simulink model "Beerbot_Simulink"  (R2020a)
settings: Solver=FixedStepAuto  StartTime=0.0  StopTime=31.5  FixedStep=0.1  RelTol=1e-3
values from neighbouring files (symbols this model uses):
  bot_wheel_distance = 0.5948    [Beerbot.m]    (also in run_Beerbot_Simulink.m)
  dual_wheel_slip_acc_thres = 1.5    [run_Beerbot_Simulink.m]
  heading_initial = Compass_Heading(1)    [run_Beerbot_Simulink.m]
  wheel_slip_detection_thres = 10.15    [run_Beerbot_Simulink.m]
  wheel_slip_detection_thres_factor = 0.8    [run_Beerbot_Simulink.m]
undefined symbols (not defined in the file or in its folder): DiscIntNeverNeededParam, theta_initial
libraries: simulink x10, dspstat3 x5, simulink_extras x2, robotmobilelib x1
settings Model: Creator=Besitzer  LastModifiedBy=Besitzer

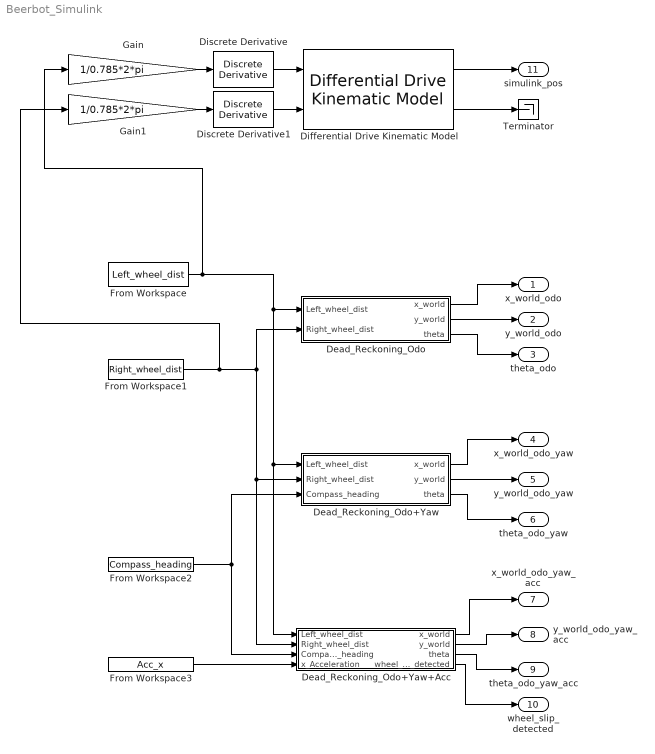
== system Beerbot_Simulink ==
  Dead_Reckoning_Odo : Subsystem
  Dead_Reckoning_Odo+Yaw : Subsystem
  Dead_Reckoning_Odo+Yaw+Acc : Subsystem
  Differential Drive Kinematic Model : robotmobilelib/Differential Drive Kinematic Model  VehicleInputs=Wheel Speeds  WheelRadius=0.1233  WheelSpeedRange=[-inf inf]  TrackWidth=0.585  InitialState=[0; 0; 0.75]  SimulateUsing=Interpreted execution
      settings: SourceProductBaseCode=RO
  Discrete Derivative : simulink/Discrete/Discrete Derivative  gainval=1.0  ICPrevScaledInput=0.0  OutMin=[]  OutMax=[]  OutDataType=fixdt(1, 16)  OutScaling=2^-10  DoSatur=off
  Discrete Derivative1 : simulink/Discrete/Discrete Derivative  gainval=1.0  ICPrevScaledInput=0.0  OutMin=[]  OutMax=[]  OutDataType=fixdt(1, 16)  OutScaling=2^-10  DoSatur=off
  From Workspace : FromWorkspace  VariableName=Left_wheel_dist
  From Workspace1 : FromWorkspace  VariableName=Right_wheel_dist
  From Workspace2 : FromWorkspace  VariableName=Compass_heading
  From Workspace3 : FromWorkspace  VariableName=Acc_x
  Gain : Gain  Gain=1/0.785*2*pi
  Gain1 : Gain  Gain=1/0.785*2*pi
  Terminator : Terminator
  x_world_odo : Outport
  y_world_odo : Outport  Port=2
  theta_odo : Outport  Port=3
  x_world_odo_yaw : Outport  Port=4
  y_world_odo_yaw : Outport  Port=5
  theta_odo_yaw : Outport  Port=6
  x_world_odo_yaw_acc : Outport  Port=7
  y_world_odo_yaw_acc : Outport  Port=8
  theta_odo_yaw_acc : Outport  Port=9
  wheel_slip_detected : Outport  Port=10
  simulink_pos : Outport  Port=11
  wires:
  From Workspace1/1 -> Gain1/1, Dead_Reckoning_Odo+Yaw+Acc/2(Right_wheel_dist), Dead_Reckoning_Odo+Yaw/2(Right_wheel_dist), Dead_Reckoning_Odo/2(Right_wheel_dist)
  Dead_Reckoning_Odo/3(theta) -> theta_odo/1
  Dead_Reckoning_Odo/1(x_world) -> x_world_odo/1
  Dead_Reckoning_Odo/2(y_world) -> y_world_odo/1
  From Workspace2/1 -> Dead_Reckoning_Odo+Yaw+Acc/3(Compass_heading), Dead_Reckoning_Odo+Yaw/3(Compass_heading)
  Dead_Reckoning_Odo+Yaw/1(x_world) -> x_world_odo_yaw/1
  Dead_Reckoning_Odo+Yaw/3(theta) -> theta_odo_yaw/1
  From Workspace3/1 -> Dead_Reckoning_Odo+Yaw+Acc/4(x_Acceleration)
  Dead_Reckoning_Odo+Yaw+Acc/3(theta) -> theta_odo_yaw_acc/1
  Dead_Reckoning_Odo+Yaw+Acc/2(y_world) -> y_world_odo_yaw_acc/1
  Dead_Reckoning_Odo+Yaw+Acc/1(x_world) -> x_world_odo_yaw_acc/1
  Dead_Reckoning_Odo+Yaw/2(y_world) -> y_world_odo_yaw/1
  Dead_Reckoning_Odo+Yaw+Acc/4(wheel_slip_detected) -> wheel_slip_detected/1
  Discrete Derivative/1 -> Differential Drive Kinematic Model/1
  Discrete Derivative1/1 -> Differential Drive Kinematic Model/2
  Differential Drive Kinematic Model/1 -> simulink_pos/1
  Differential Drive Kinematic Model/2 -> Terminator/1
  From Workspace/1 -> Gain/1, Dead_Reckoning_Odo/1(Left_wheel_dist), Dead_Reckoning_Odo+Yaw+Acc/1(Left_wheel_dist), Dead_Reckoning_Odo+Yaw/1(Left_wheel_dist)
  Gain/1 -> Discrete Derivative/1
  Gain1/1 -> Discrete Derivative1/1

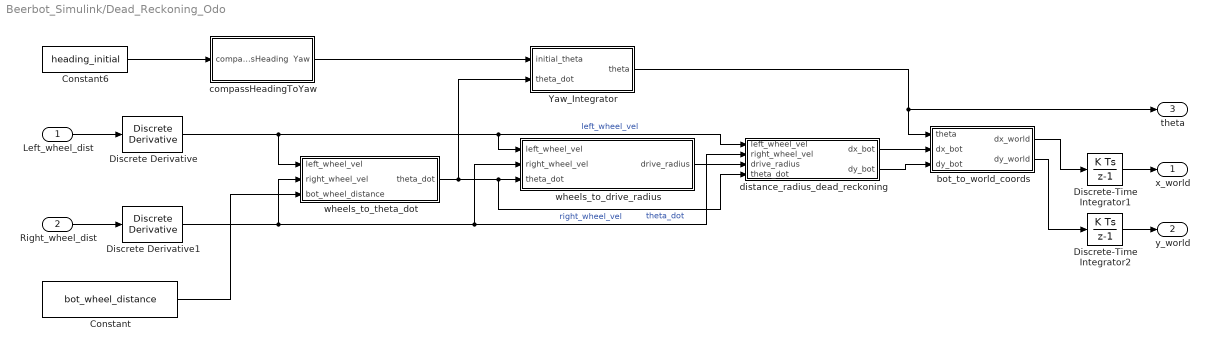
== system Beerbot_Simulink/Dead_Reckoning_Odo ==
  Left_wheel_dist : Inport
  Right_wheel_dist : Inport  Port=2
  Constant : Constant  Value=bot_wheel_distance
  Constant6 : Constant  Value=heading_initial
  Discrete Derivative : simulink/Discrete/Discrete Derivative  gainval=1.0  ICPrevScaledInput=0.0  OutMin=[]  OutMax=[]  OutDataType=fixdt(1, 16)  OutScaling=2^-10  DoSatur=off
      settings: AttributesFormatString=%<Name>
  Discrete Derivative1 : simulink/Discrete/Discrete Derivative  gainval=1.0  ICPrevScaledInput=0.0  OutMin=[]  OutMax=[]  OutDataType=fixdt(1, 16)  OutScaling=2^-10  DoSatur=off
      settings: AttributesFormatString=%<Name>
  Discrete-Time Integrator1 : DiscreteIntegrator  SampleTime=-1  ICPrevOutput=DiscIntNeverNeededParam  ICPrevScaledInput=DiscIntNeverNeededParam
      settings: AttributesFormatString=%<Name>
  Discrete-Time Integrator2 : DiscreteIntegrator  SampleTime=-1  ICPrevOutput=DiscIntNeverNeededParam  ICPrevScaledInput=DiscIntNeverNeededParam
      settings: AttributesFormatString=%<Name>
  Yaw_Integrator : Subsystem
  bot_to_world_coords : Subsystem
  compassHeadingToYaw : Subsystem
  distance_radius_dead_reckoning : Subsystem
  wheels_to_drive_radius : Subsystem
  wheels_to_theta_dot : Subsystem
  x_world : Outport
  y_world : Outport  Port=2
  theta : Outport  Port=3
  wires:
  Left_wheel_dist/1 -> Discrete Derivative/1
  Right_wheel_dist/1 -> Discrete Derivative1/1
  Discrete Derivative1/1 -> wheels_to_theta_dot/2(right_wheel_vel), wheels_to_drive_radius/2(right_wheel_vel), distance_radius_dead_reckoning/2(right_wheel_vel)  "right_wheel_vel"
  Discrete Derivative/1 -> distance_radius_dead_reckoning/1(left_wheel_vel), wheels_to_drive_radius/1(left_wheel_vel), wheels_to_theta_dot/1(left_wheel_vel)  "left_wheel_vel"
  wheels_to_theta_dot/1(theta_dot) -> distance_radius_dead_reckoning/4(theta_dot), wheels_to_drive_radius/3(theta_dot), Yaw_Integrator/2(theta_dot)  "theta_dot"
  Yaw_Integrator/1(theta) -> theta/1, bot_to_world_coords/1(theta)
  Discrete-Time Integrator1/1 -> x_world/1
  Discrete-Time Integrator2/1 -> y_world/1
  compassHeadingToYaw/1(Yaw) -> Yaw_Integrator/1(initial_theta)
  Constant6/1 -> compassHeadingToYaw/1(compassHeading)
  bot_to_world_coords/1(dx_world) -> Discrete-Time Integrator1/1
  bot_to_world_coords/2(dy_world) -> Discrete-Time Integrator2/1
  Constant/1 -> wheels_to_theta_dot/3(bot_wheel_distance)
  wheels_to_drive_radius/1(drive_radius) -> distance_radius_dead_reckoning/3(drive_radius)
  distance_radius_dead_reckoning/1(dx_bot) -> bot_to_world_coords/2(dx_bot)
  distance_radius_dead_reckoning/2(dy_bot) -> bot_to_world_coords/3(dy_bot)

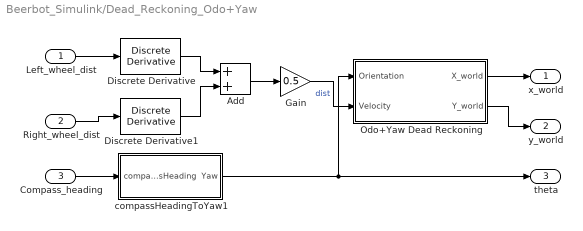
== system Beerbot_Simulink/Dead_Reckoning_Odo+Yaw ==
  Left_wheel_dist : Inport
  Right_wheel_dist : Inport  Port=2
  Compass_heading : Inport  Port=3
  Add : Sum
  Discrete Derivative : simulink/Discrete/Discrete Derivative  gainval=1.0  ICPrevScaledInput=0.0  OutMin=[]  OutMax=[]  OutDataType=fixdt(1, 16)  OutScaling=2^-10  DoSatur=off
  Discrete Derivative1 : simulink/Discrete/Discrete Derivative  gainval=1.0  ICPrevScaledInput=0.0  OutMin=[]  OutMax=[]  OutDataType=fixdt(1, 16)  OutScaling=2^-10  DoSatur=off
  Gain : Gain  Gain=0.5
  Odo+Yaw Dead Reckoning : Subsystem
  compassHeadingToYaw1 : Subsystem
  x_world : Outport
  y_world : Outport  Port=2
  theta : Outport  Port=3
  wires:
  Add/1 -> Gain/1
  Compass_heading/1 -> compassHeadingToYaw1/1(compassHeading)
  compassHeadingToYaw1/1(Yaw) -> Odo+Yaw Dead Reckoning/1(Orientation), theta/1
  Left_wheel_dist/1 -> Discrete Derivative/1
  Discrete Derivative/1 -> Add/1
  Discrete Derivative1/1 -> Add/2
  Right_wheel_dist/1 -> Discrete Derivative1/1
  Gain/1 -> Odo+Yaw Dead Reckoning/2(Velocity)  "dist"
  Odo+Yaw Dead Reckoning/1(X_world) -> x_world/1
  Odo+Yaw Dead Reckoning/2(Y_world) -> y_world/1

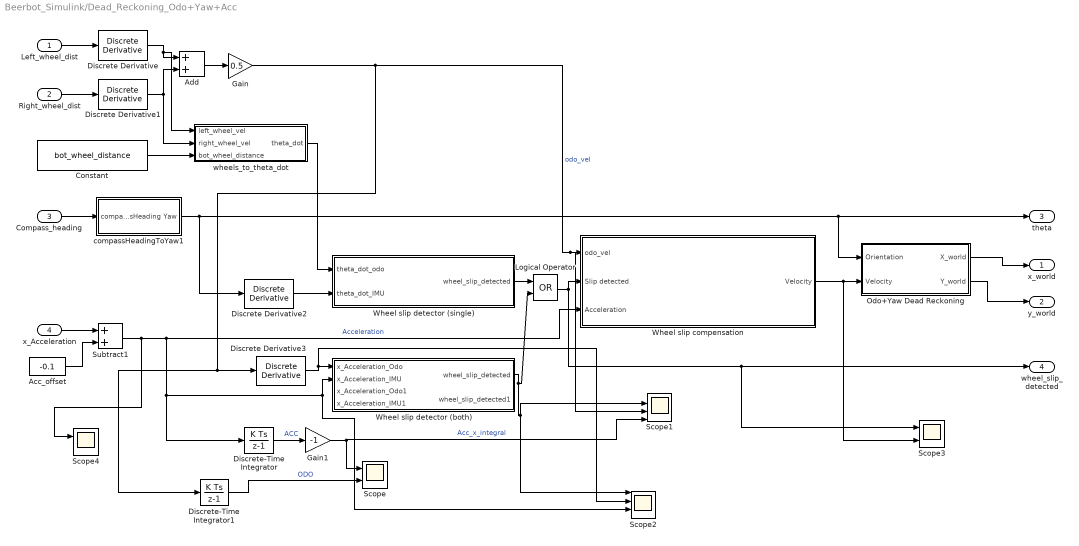
== system Beerbot_Simulink/Dead_Reckoning_Odo+Yaw+Acc ==
  Left_wheel_dist : Inport
  Right_wheel_dist : Inport  Port=2
  Compass_heading : Inport  Port=3
  x_Acceleration : Inport  Port=4
  Acc_offset : Constant  Value=-0.1
  Add : Sum
  Constant : Constant  Value=bot_wheel_distance
  Discrete Derivative{,1..3} (4 alike) : simulink/Discrete/Discrete Derivative  gainval=1.0  ICPrevScaledInput=0.0  OutMin=[]  OutMax=[]  OutDataType=fixdt(1, 16)  OutScaling=2^-10  DoSatur=off
  Discrete-Time Integrator : DiscreteIntegrator  SampleTime=-1  ICPrevOutput=DiscIntNeverNeededParam  ICPrevScaledInput=DiscIntNeverNeededParam
  Discrete-Time Integrator1 : DiscreteIntegrator  SampleTime=-1  ICPrevOutput=DiscIntNeverNeededParam  ICPrevScaledInput=DiscIntNeverNeededParam
  Gain : Gain  Gain=0.5
  Gain1 : Gain  Gain=-1
  Logical Operator : Logic  Operator=OR  AllPortsSameDT=off  OutDataTypeStr=boolean
  Odo+Yaw Dead Reckoning : Subsystem
  Scope : Scope  NumInputPorts=2
  Scope1 : Scope  NumInputPorts=4
  Scope2 : Scope  NumInputPorts=4
  Scope3 : Scope  NumInputPorts=2
  Scope4 : Scope  NumInputPorts=2
  Subtract1 : Sum
  Wheel slip compensation : Subsystem
  Wheel slip detector (both) : Subsystem
  Wheel slip detector (single) : Subsystem
  compassHeadingToYaw1 : Subsystem
  wheels_to_theta_dot : Subsystem
  x_world : Outport
  y_world : Outport  Port=2
  theta : Outport  Port=3
  wheel_slip_detected : Outport  Port=4  OutDataTypeStr=boolean  LockScale=on
  wires:
  Add/1 -> Gain/1
  Compass_heading/1 -> compassHeadingToYaw1/1(compassHeading)
  compassHeadingToYaw1/1(Yaw) -> Discrete Derivative2/1, Odo+Yaw Dead Reckoning/1(Orientation), theta/1
  Left_wheel_dist/1 -> Discrete Derivative/1
  Discrete Derivative/1 -> wheels_to_theta_dot/1(left_wheel_vel), Add/1
  Discrete Derivative1/1 -> wheels_to_theta_dot/2(right_wheel_vel), Add/2
  Right_wheel_dist/1 -> Discrete Derivative1/1
  x_Acceleration/1 -> Subtract1/1
  Constant/1 -> wheels_to_theta_dot/3(bot_wheel_distance)
  wheels_to_theta_dot/1(theta_dot) -> Wheel slip detector (single)/1(theta_dot_odo)
  Acc_offset/1 -> Subtract1/2
  Logical Operator/1 -> Wheel slip compensation/2(Slip detected), Scope3/1, wheel_slip_detected/1
  Discrete Derivative2/1 -> Wheel slip detector (single)/2(theta_dot_IMU)
  Gain/1 -> Discrete Derivative3/1, Discrete-Time Integrator1/1, Scope1/3, Wheel slip compensation/1(odo_vel)  "odo_vel"
  Subtract1/1 -> Scope4/1, Wheel slip compensation/3(Acceleration), Discrete-Time Integrator/1, Scope2/3, Wheel slip detector (both)/2(x_Acceleration_IMU)  "Acceleration"
  Odo+Yaw Dead Reckoning/2(Y_world) -> y_world/1
  Odo+Yaw Dead Reckoning/1(X_world) -> x_world/1
  Wheel slip compensation/1(Velocity) -> Scope3/2, Odo+Yaw Dead Reckoning/2(Velocity)
  Wheel slip detector (single)/1(wheel_slip_detected) -> Logical Operator/1
  Wheel slip detector (both)/1(wheel_slip_detected) -> Scope2/1, Scope1/2, Logical Operator/2
  Discrete Derivative3/1 -> Scope2/2, Wheel slip detector (both)/1(x_Acceleration_Odo)
  Discrete-Time Integrator/1 -> Gain1/1  "ACC"
  Discrete-Time Integrator1/1 -> Scope/2  "ODO"
  Gain1/1 -> Scope/1, Scope1/4  "Acc_x_integral"

== system Beerbot_Simulink/Dead_Reckoning_Odo/Yaw_Integrator ==
  initial_theta : Inport
  theta_dot : Inport  Port=2
  Constant5 : Constant  Value=2*pi
  Discrete-Time Integrator : DiscreteIntegrator  InitialConditionSource=external  InitialCondition=theta_initial  SampleTime=-1  ICPrevOutput=DiscIntNeverNeededParam  ICPrevScaledInput=DiscIntNeverNeededParam
      settings: AttributesFormatString=%<Name>
  Mod : Math  Operator=mod  SaturateOnIntegerOverflow=on
  theta : Outport
  wires:
  Constant5/1 -> Mod/2
  Discrete-Time Integrator/1 -> Mod/1
  initial_theta/1 -> Discrete-Time Integrator/2
  theta_dot/1 -> Discrete-Time Integrator/1
  Mod/1 -> theta/1

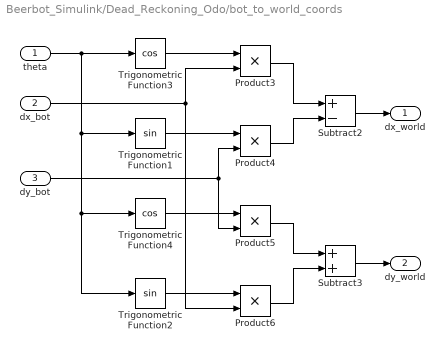
== system Beerbot_Simulink/Dead_Reckoning_Odo/bot_to_world_coords ==
  theta : Inport
  dx_bot : Inport  Port=2
  dy_bot : Inport  Port=3
  Product{3..6} (4 alike) : Product
  Subtract2 : Sum  Inputs=+-
  Subtract3 : Sum
  Trigonometric Function1 : Trigonometry
  Trigonometric Function2 : Trigonometry
  Trigonometric Function3 : Trigonometry  Operator=cos
  Trigonometric Function4 : Trigonometry  Operator=cos
  dx_world : Outport
  dy_world : Outport  Port=2
  wires:
  Subtract2/1 -> dx_world/1
  Subtract3/1 -> dy_world/1
  Trigonometric Function1/1 -> Product4/1
  Trigonometric Function3/1 -> Product3/1
  theta/1 -> Trigonometric Function3/1, Trigonometric Function2/1, Trigonometric Function4/1, Trigonometric Function1/1
  dx_bot/1 -> Product3/2, Product6/2
  Product5/1 -> Subtract3/1
  Product6/1 -> Subtract3/2
  dy_bot/1 -> Product5/2, Product4/2
  Product3/1 -> Subtract2/1
  Product4/1 -> Subtract2/2
  Trigonometric Function2/1 -> Product6/1
  Trigonometric Function4/1 -> Product5/1

== system Beerbot_Simulink/Dead_Reckoning_Odo/compassHeadingToYaw ==
  compassHeading : Inport
  Add : Sum
  Constant : Constant  Value=2*pi
  Constant1 : Constant  Value=pi/2
  Mod : Math  Operator=mod  SaturateOnIntegerOverflow=on
  Subtract : Sum  Inputs=+-
  Yaw : Outport
  wires:
  Constant/1 -> Mod/2, Subtract/1
  compassHeading/1 -> Subtract/2
  Subtract/1 -> Add/1
  Constant1/1 -> Add/2
  Add/1 -> Mod/1
  Mod/1 -> Yaw/1

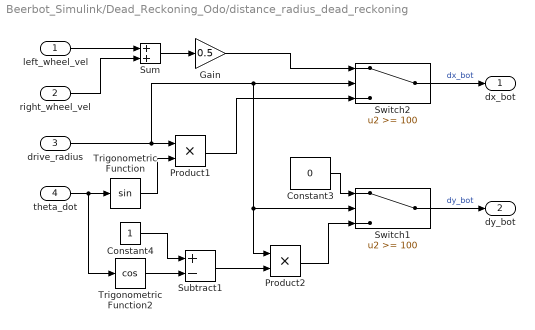
== system Beerbot_Simulink/Dead_Reckoning_Odo/distance_radius_dead_reckoning ==
  left_wheel_vel : Inport
  right_wheel_vel : Inport  Port=2
  drive_radius : Inport  Port=3
  theta_dot : Inport  Port=4
  Constant3 : Constant  Value=0
  Constant4 : Constant
  Gain : Gain  Gain=0.5
  Product1 : Product
  Product2 : Product
  Subtract1 : Sum  Inputs=+-
  Sum : Sum
  Switch1 : Switch  Threshold=100
  Switch2 : Switch  Threshold=100
  Trigonometric Function : Trigonometry
  Trigonometric Function2 : Trigonometry  Operator=cos
  dx_bot : Outport
  dy_bot : Outport  Port=2
  wires:
  left_wheel_vel/1 -> Sum/1
  Switch2/1 -> dx_bot/1  "dx_bot"
  Trigonometric Function/1 -> Product1/2
  right_wheel_vel/1 -> Sum/2
  Trigonometric Function2/1 -> Subtract1/2
  Switch1/1 -> dy_bot/1  "dy_bot"
  drive_radius/1 -> Product2/1, Switch1/2, Switch2/2, Product1/1
  Subtract1/1 -> Product2/2
  Product1/1 -> Switch2/3
  Product2/1 -> Switch1/3
  theta_dot/1 -> Trigonometric Function/1, Trigonometric Function2/1
  Constant3/1 -> Switch1/1
  Sum/1 -> Gain/1
  Gain/1 -> Switch2/1
  Constant4/1 -> Subtract1/1

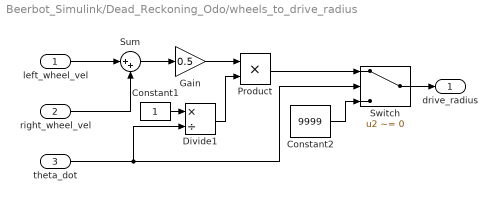
== system Beerbot_Simulink/Dead_Reckoning_Odo/wheels_to_drive_radius ==
  left_wheel_vel : Inport
  right_wheel_vel : Inport  Port=2
  theta_dot : Inport  Port=3
  Constant1 : Constant
  Constant2 : Constant  Value=9999
  Divide1 : Product  Inputs=*/
  Gain : Gain  Gain=0.5
  Product : Product
  Sum : Sum  Inputs=|++
  Switch : Switch  Criteria=u2 ~= 0
  drive_radius : Outport
  wires:
  right_wheel_vel/1 -> Sum/2
  theta_dot/1 -> Switch/2, Divide1/2
  Sum/1 -> Gain/1
  Divide1/1 -> Product/2
  Gain/1 -> Product/1
  Constant1/1 -> Divide1/1
  left_wheel_vel/1 -> Sum/1
  Constant2/1 -> Switch/3
  Product/1 -> Switch/1
  Switch/1 -> drive_radius/1

== system Beerbot_Simulink/Dead_Reckoning_Odo/wheels_to_theta_dot ==
  left_wheel_vel : Inport
  right_wheel_vel : Inport  Port=2
  bot_wheel_distance : Inport  Port=3
  Divide : Product  Inputs=*/
  Subtract : Sum  Inputs=-+
  theta_dot : Outport
  wires:
  left_wheel_vel/1 -> Subtract/1
  Divide/1 -> theta_dot/1
  right_wheel_vel/1 -> Subtract/2
  Subtract/1 -> Divide/1
  bot_wheel_distance/1 -> Divide/2

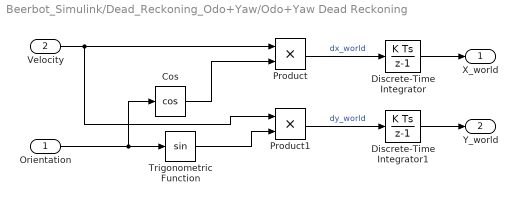
== system Beerbot_Simulink/Dead_Reckoning_Odo+Yaw/Odo+Yaw Dead Reckoning ==
  Orientation : Inport
  Velocity : Inport  Port=2
  Cos : Trigonometry  Operator=cos
  Discrete-Time Integrator : DiscreteIntegrator  SampleTime=-1  ICPrevOutput=DiscIntNeverNeededParam  ICPrevScaledInput=DiscIntNeverNeededParam
  Discrete-Time Integrator1 : DiscreteIntegrator  SampleTime=-1  ICPrevOutput=DiscIntNeverNeededParam  ICPrevScaledInput=DiscIntNeverNeededParam
  Product : Product
  Product1 : Product
  Trigonometric Function : Trigonometry
  X_world : Outport
  Y_world : Outport  Port=2
  wires:
  Cos/1 -> Product/2
  Product/1 -> Discrete-Time Integrator/1  "dx_world"
  Trigonometric Function/1 -> Product1/2
  Velocity/1 -> Product1/1, Product/1
  Orientation/1 -> Cos/1, Trigonometric Function/1
  Discrete-Time Integrator1/1 -> Y_world/1
  Product1/1 -> Discrete-Time Integrator1/1  "dy_world"
  Discrete-Time Integrator/1 -> X_world/1

== system Beerbot_Simulink/Dead_Reckoning_Odo+Yaw/compassHeadingToYaw1 ==
  compassHeading : Inport
  Add : Sum
  Constant : Constant  Value=2*pi
  Constant1 : Constant  Value=pi/2
  Mod : Math  Operator=mod  SaturateOnIntegerOverflow=on
  Subtract : Sum  Inputs=+-
  Yaw : Outport
  wires:
  Constant/1 -> Mod/2, Subtract/1
  compassHeading/1 -> Subtract/2
  Subtract/1 -> Add/1
  Constant1/1 -> Add/2
  Add/1 -> Mod/1
  Mod/1 -> Yaw/1

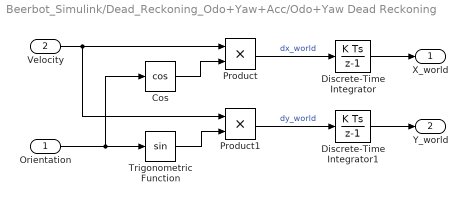
== system Beerbot_Simulink/Dead_Reckoning_Odo+Yaw+Acc/Odo+Yaw Dead Reckoning ==
  Orientation : Inport
  Velocity : Inport  Port=2
  Cos : Trigonometry  Operator=cos
  Discrete-Time Integrator : DiscreteIntegrator  SampleTime=-1  ICPrevOutput=DiscIntNeverNeededParam  ICPrevScaledInput=DiscIntNeverNeededParam
  Discrete-Time Integrator1 : DiscreteIntegrator  SampleTime=-1  ICPrevOutput=DiscIntNeverNeededParam  ICPrevScaledInput=DiscIntNeverNeededParam
  Product : Product
  Product1 : Product
  Trigonometric Function : Trigonometry
  X_world : Outport
  Y_world : Outport  Port=2
  wires:
  Cos/1 -> Product/2
  Product/1 -> Discrete-Time Integrator/1  "dx_world"
  Trigonometric Function/1 -> Product1/2
  Velocity/1 -> Product1/1, Product/1
  Orientation/1 -> Cos/1, Trigonometric Function/1
  Discrete-Time Integrator1/1 -> Y_world/1
  Product1/1 -> Discrete-Time Integrator1/1  "dy_world"
  Discrete-Time Integrator/1 -> X_world/1

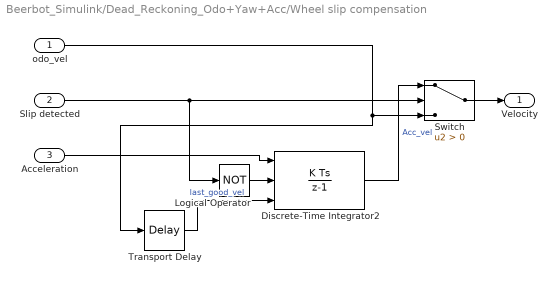
== system Beerbot_Simulink/Dead_Reckoning_Odo+Yaw+Acc/Wheel slip compensation ==
  odo_vel : Inport
  Slip detected : Inport  Port=2
  Acceleration : Inport  Port=3
  Discrete-Time Integrator2 : DiscreteIntegrator  ExternalReset=level  InitialConditionSource=external  SampleTime=-1  ICPrevOutput=DiscIntNeverNeededParam  ICPrevScaledInput=DiscIntNeverNeededParam
  Logical Operator : Logic  Operator=NOT  AllPortsSameDT=off  OutDataTypeStr=boolean
  Switch : Switch  Criteria=u2 > Threshold
  Transport Delay : TransportDelay  DelayTime=0.5
  Velocity : Outport
  wires:
  odo_vel/1 -> Transport Delay/1, Switch/3
  Switch/1 -> Velocity/1
  Logical Operator/1 -> Discrete-Time Integrator2/2
  Discrete-Time Integrator2/1 -> Switch/1  "Acc_vel"
  Transport Delay/1 -> Discrete-Time Integrator2/3  "last_good_vel"
  Acceleration/1 -> Discrete-Time Integrator2/1
  Slip detected/1 -> Switch/2, Logical Operator/1

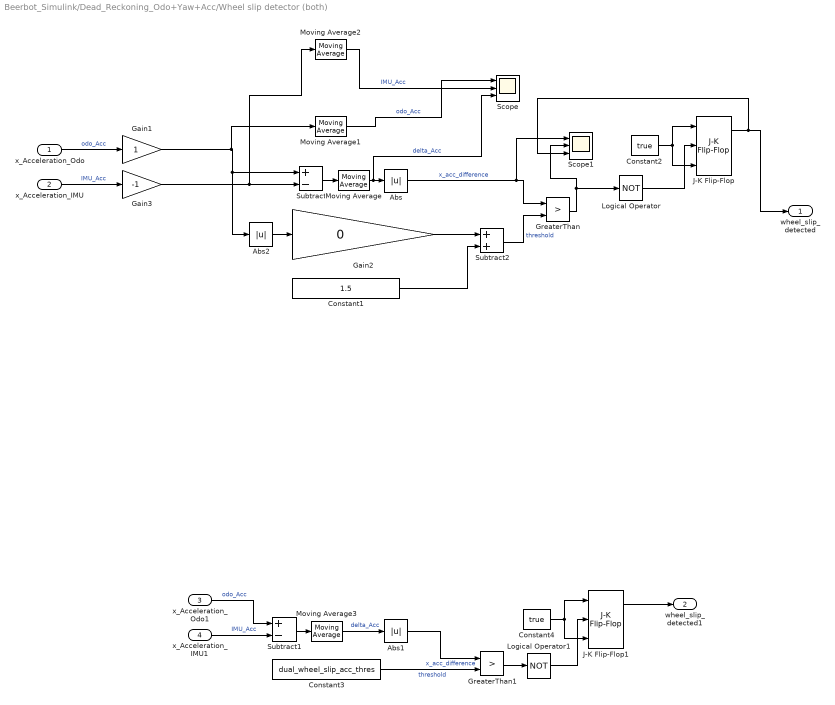
== system Beerbot_Simulink/Dead_Reckoning_Odo+Yaw+Acc/Wheel slip detector (both) ==
  x_Acceleration_Odo : Inport
  x_Acceleration_IMU : Inport  Port=2
  x_Acceleration_Odo1 : Inport  Port=3
  x_Acceleration_IMU1 : Inport  Port=4
  Abs : Abs
  Abs1 : Abs
  Abs2 : Abs
  Constant1 : Constant  Value=1.5
  Constant2 : Constant  Value=true
  Constant3 : Constant  Value=dual_wheel_slip_acc_thres
  Constant4 : Constant  Value=true
  Gain1 : Gain
  Gain2 : Gain  Gain=0
  Gain3 : Gain  Gain=-1
  GreaterThan : RelationalOperator  Operator=>  OutDataTypeStr=boolean  RndMeth=Simplest
  GreaterThan1 : RelationalOperator  Operator=>  OutDataTypeStr=boolean  RndMeth=Simplest
  J-K Flip-Flop : simulink_extras/Flip Flops/J-K Flip-Flop  initial_condition=0
  J-K Flip-Flop1 : simulink_extras/Flip Flops/J-K Flip-Flop  initial_condition=0
  Logical Operator : Logic  Operator=NOT  AllPortsSameDT=off  OutDataTypeStr=boolean
  Logical Operator1 : Logic  Operator=NOT  AllPortsSameDT=off  OutDataTypeStr=boolean
  Moving Average : dspstat3/Moving Average  Method=Sliding window  ForgettingFactorPort=off  SpecifyWindowLength=on  WindowLength=5  ForgettingFactor=0.9  SimulateUsing=Code generation
  Moving Average1 : dspstat3/Moving Average  Method=Sliding window  ForgettingFactorPort=off  SpecifyWindowLength=on  WindowLength=2  ForgettingFactor=0.9  SimulateUsing=Code generation
  Moving Average2 : dspstat3/Moving Average  Method=Sliding window  ForgettingFactorPort=off  SpecifyWindowLength=on  WindowLength=2  ForgettingFactor=0.9  SimulateUsing=Code generation
  Moving Average3 : dspstat3/Moving Average  Method=Sliding window  ForgettingFactorPort=off  SpecifyWindowLength=on  WindowLength=5  ForgettingFactor=0.9  SimulateUsing=Code generation
  Scope : Scope  NumInputPorts=3
  Scope1 : Scope  NumInputPorts=3
  Subtract : Sum  Inputs=+-
  Subtract1 : Sum  Inputs=+-
  Subtract2 : Sum
  wheel_slip_detected : Outport
  wheel_slip_detected1 : Outport  Port=2
  wires:
  Moving Average/1 -> Scope/3, Abs/1  "delta_Acc"
  Abs2/1 -> Gain2/1
  Subtract2/1 -> GreaterThan/2  "threshold"
  Gain2/1 -> Subtract2/1
  Subtract/1 -> Moving Average/1
  Constant1/1 -> Subtract2/2
  Abs/1 -> Scope1/1, GreaterThan/1  "x_acc_difference"
  GreaterThan/1 -> Logical Operator/1, Scope1/2
  x_Acceleration_Odo/1 -> Gain1/1  "odo_Acc"
  x_Acceleration_IMU/1 -> Gain3/1  "IMU_Acc"
  Gain1/1 -> Moving Average1/1, Subtract/1, Abs2/1
  Moving Average2/1 -> Scope/2  "IMU_Acc"
  Moving Average1/1 -> Scope/1  "odo_Acc"
  Gain3/1 -> Moving Average2/1, Subtract/2
  Constant2/1 -> J-K Flip-Flop/1, J-K Flip-Flop/3
  J-K Flip-Flop/1 -> Scope1/3, wheel_slip_detected/1
  Logical Operator/1 -> J-K Flip-Flop/2
  J-K Flip-Flop1/1 -> wheel_slip_detected1/1
  Constant4/1 -> J-K Flip-Flop1/1, J-K Flip-Flop1/3
  Logical Operator1/1 -> J-K Flip-Flop1/2
  Abs1/1 -> GreaterThan1/1  "x_acc_difference"
  Subtract1/1 -> Moving Average3/1
  GreaterThan1/1 -> Logical Operator1/1
  x_Acceleration_IMU1/1 -> Subtract1/2  "IMU_Acc"
  Moving Average3/1 -> Abs1/1  "delta_Acc"
  x_Acceleration_Odo1/1 -> Subtract1/1  "odo_Acc"
  Constant3/1 -> GreaterThan1/2  "threshold"

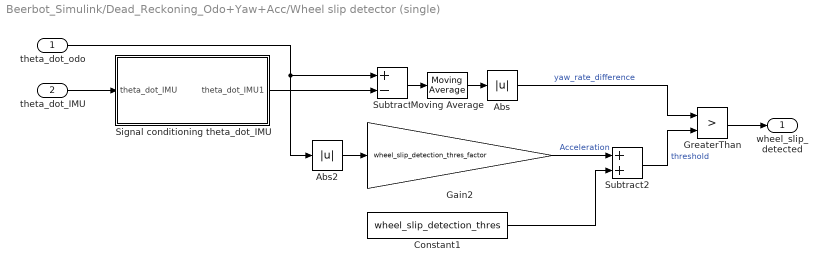
== system Beerbot_Simulink/Dead_Reckoning_Odo+Yaw+Acc/Wheel slip detector (single) ==
  theta_dot_odo : Inport
  theta_dot_IMU : Inport  Port=2
  Abs : Abs
  Abs2 : Abs
  Constant1 : Constant  Value=wheel_slip_detection_thres
  Gain2 : Gain  Gain=wheel_slip_detection_thres_factor
  GreaterThan : RelationalOperator  Operator=>  OutDataTypeStr=boolean  RndMeth=Simplest
  Moving Average : dspstat3/Moving Average  Method=Sliding window  ForgettingFactorPort=off  SpecifyWindowLength=on  WindowLength=5  ForgettingFactor=0.9  SimulateUsing=Code generation
  Signal conditioning theta_dot_IMU : Subsystem
  Subtract : Sum  Inputs=+-
  Subtract2 : Sum
  wheel_slip_detected : Outport
  wires:
  Moving Average/1 -> Abs/1
  theta_dot_odo/1 -> Subtract/1, Abs2/1
  Abs2/1 -> Gain2/1
  Subtract2/1 -> GreaterThan/2  "threshold"
  Gain2/1 -> Subtract2/1  "Acceleration"
  Subtract/1 -> Moving Average/1
  Constant1/1 -> Subtract2/2
  Abs/1 -> GreaterThan/1  "yaw_rate_difference"
  GreaterThan/1 -> wheel_slip_detected/1
  theta_dot_IMU/1 -> Signal conditioning theta_dot_IMU/1(theta_dot_IMU)
  Signal conditioning theta_dot_IMU/1(theta_dot_IMU1) -> Subtract/2

== system Beerbot_Simulink/Dead_Reckoning_Odo+Yaw+Acc/compassHeadingToYaw1 ==
  compassHeading : Inport
  Add : Sum
  Constant : Constant  Value=2*pi
  Constant1 : Constant  Value=pi/2
  Mod : Math  Operator=mod  SaturateOnIntegerOverflow=on
  Subtract : Sum  Inputs=+-
  Yaw : Outport
  wires:
  Constant/1 -> Mod/2, Subtract/1
  compassHeading/1 -> Subtract/2
  Subtract/1 -> Add/1
  Constant1/1 -> Add/2
  Add/1 -> Mod/1
  Mod/1 -> Yaw/1

== system Beerbot_Simulink/Dead_Reckoning_Odo+Yaw+Acc/wheels_to_theta_dot ==
  left_wheel_vel : Inport
  right_wheel_vel : Inport  Port=2
  bot_wheel_distance : Inport  Port=3
  Divide : Product  Inputs=*/
  Subtract : Sum  Inputs=-+
  theta_dot : Outport
  wires:
  left_wheel_vel/1 -> Subtract/1
  Divide/1 -> theta_dot/1
  right_wheel_vel/1 -> Subtract/2
  Subtract/1 -> Divide/1
  bot_wheel_distance/1 -> Divide/2

== system Beerbot_Simulink/Dead_Reckoning_Odo+Yaw+Acc/Wheel slip detector (single)/Signal conditioning theta_dot_IMU ==
  note: Suppress peaks due to 2*Pi <-> 0 radians differential
  theta_dot_IMU : Inport
  Abs1 : Abs
  Constant2 : Constant  Value=0
  Switch1 : Switch  Criteria=u2 > Threshold  Threshold=2
  theta_dot_IMU1 : Outport
  wires:
  theta_dot_IMU/1 -> Abs1/1, Switch1/3
  Switch1/1 -> theta_dot_IMU1/1  "theta_dot_IMU"
  Constant2/1 -> Switch1/1
  Abs1/1 -> Switch1/2
